simulink subsystem "Ledss"  (R2023b)
settings: Solver=VariableStepAuto  StartTime=0.0  StopTime=10.0  RelTol=1e-3
libraries: simulink x4, arduinolib x3
settings Model: Creator=marqu  LastModifiedBy=marqu

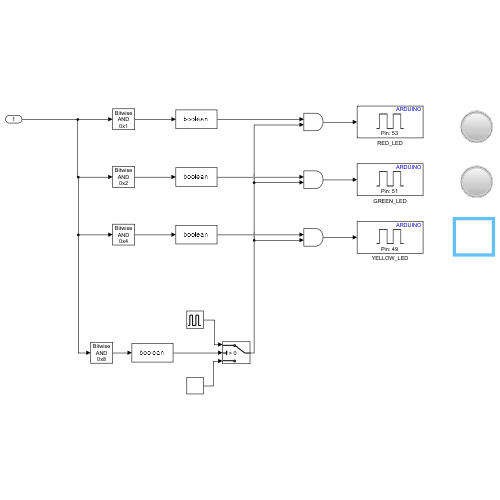
[thumbnail: Simulink's stored preview of the top-level diagram]
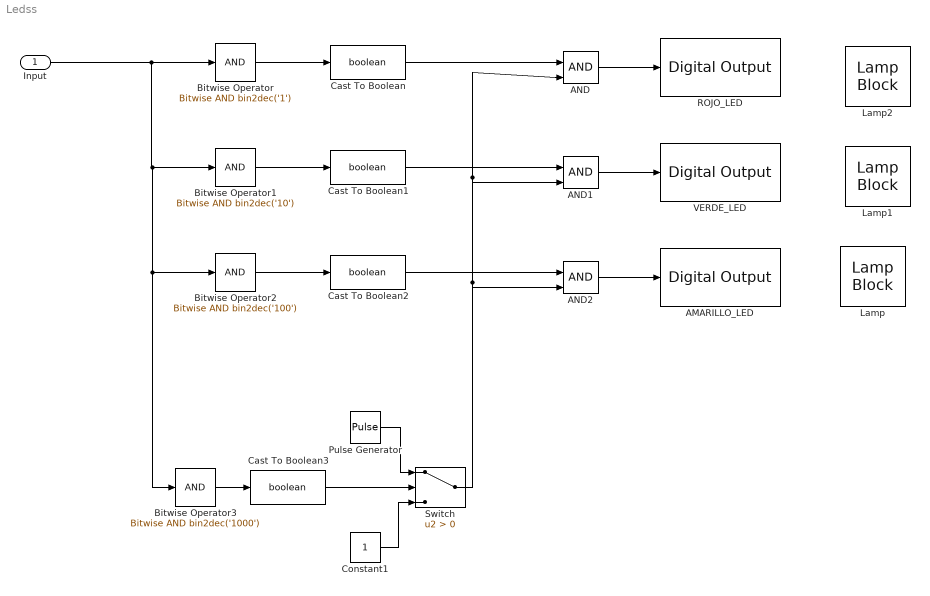
== system Ledss ==
  Input : Inport
  AMARILLO_LED : arduinolib/Digital Output  pinNumber=49  Direction=output  blockPlatform=arduino
  AND : Logic  IconShape=distinctive  AllPortsSameDT=off  OutDataTypeStr=boolean
  AND1 : Logic  IconShape=distinctive  AllPortsSameDT=off  OutDataTypeStr=boolean
  AND2 : Logic  IconShape=distinctive  AllPortsSameDT=off  OutDataTypeStr=boolean
  Bitwise Operator : simulink/Logic and Bit Operations/Bitwise Operator  logicop=AND  UseBitMask=on  BitMask=bin2dec('1')  BitMaskRealWorld=Stored Integer
  Bitwise Operator1 : simulink/Logic and Bit Operations/Bitwise Operator  logicop=AND  UseBitMask=on  BitMask=bin2dec('10')  BitMaskRealWorld=Stored Integer
  Bitwise Operator2 : simulink/Logic and Bit Operations/Bitwise Operator  logicop=AND  UseBitMask=on  BitMask=bin2dec('100')  BitMaskRealWorld=Stored Integer
  Bitwise Operator3 : simulink/Logic and Bit Operations/Bitwise Operator  logicop=AND  UseBitMask=on  BitMask=bin2dec('1000')  BitMaskRealWorld=Stored Integer
  Cast To Boolean{,1..3} (4 alike) : DataTypeConversion  OutDataTypeStr=boolean  SaturateOnIntegerOverflow=off  RndMeth=Floor
  Constant1 : Constant
  Lamp : LampBlock  LabelPosition=Hide
  Lamp1 : LampBlock  LabelPosition=Hide
  Lamp2 : LampBlock  LabelPosition=Hide
  Pulse Generator : DiscretePulseGenerator  PulseType=Time based  Period=0.5  PulseWidth=50
  ROJO_LED : arduinolib/Digital Output  pinNumber=53  Direction=output  blockPlatform=arduino
  Switch : Switch  Criteria=u2 > Threshold  SaturateOnIntegerOverflow=off  InputSameDT=off
  VERDE_LED : arduinolib/Digital Output  pinNumber=51  Direction=output  blockPlatform=arduino
  wires:
  Pulse Generator/1 -> Switch/1
  Input/1 -> Bitwise Operator3/1, Bitwise Operator2/1, Bitwise Operator1/1, Bitwise Operator/1
  AND2/1 -> AMARILLO_LED/1
  Bitwise Operator3/1 -> Cast To Boolean3/1
  Cast To Boolean1/1 -> AND1/1
  Bitwise Operator/1 -> Cast To Boolean/1
  Cast To Boolean3/1 -> Switch/2
  Switch/1 -> AND/2, AND1/2, AND2/2
  Bitwise Operator1/1 -> Cast To Boolean1/1
  Cast To Boolean2/1 -> AND2/1
  Bitwise Operator2/1 -> Cast To Boolean2/1
  Cast To Boolean/1 -> AND/1
  Constant1/1 -> Switch/3
  AND/1 -> ROJO_LED/1
  AND1/1 -> VERDE_LED/1
